simulink model "PubIfDecisionLSM_MDL"  (R2020b)
settings: configuration reference "DspaceConfig" (kept outside this file)
PostLoadFcn:
  | if any(exist('dsrtsu_mdlpostloadfcn', 'file') ~= 0), dsrtsu_mdlpostloadfcn('Execute', bdroot); end
InitFcn:
  | , if any(exist('rtifpga_mdlclblib', 'file') ~= 0), rtifpga_mdlclblib('Init', bdroot); end,
  | , if any(exist('dsmpb_private', 'file') ~= 0), dsmpb_private('dsmpb_mdlclblib', 'Init', bdroot); end,
values from neighbouring files (symbols this model uses):
  P_LSM_ALC_Enable = 0.0    [LSM_Parameter.sldd]
  P_LSM_AwayEdge_offset = 0.1    [LSM_Parameter.sldd]
  P_LSM_CentValidErr = 1.0    [LSM_Parameter.sldd]
  P_LSM_DOP_C0_EN_Limit = 0.8    [LSM_Parameter.sldd]
  P_LSM_DOP_C0_out_Limit = 2.0    [LSM_Parameter.sldd]
  P_LSM_DOP_C1_EN_Limit : value not decoded    [LSM_Parameter.sldd]
  P_LSM_DOP_C1_out_Limit : value not decoded    [LSM_Parameter.sldd]
  P_LSM_DOP_C1AndC2_Lim_X : value not decoded    [LSM_Parameter.sldd]
  P_LSM_DOP_C2_EN_Limit : value not decoded    [LSM_Parameter.sldd]
  P_LSM_DOP_C2_out_Limit : value not decoded    [LSM_Parameter.sldd]
  P_LSM_DOP_In_Pre2Dop_Dis = 1.0    [LSM_Parameter.sldd]
  P_LSM_DOP_Out_Pre2Dop_Dis = 2.0    [LSM_Parameter.sldd]
  P_LSM_DOP_PreDis_X : value not decoded    [LSM_Parameter.sldd]
  P_LSM_DOP_PreDis_Y : value not decoded    [LSM_Parameter.sldd]
  P_LSM_DOPEnableSW = 1.0    [LSM_Parameter.sldd]
  P_LSM_DOPValid_CheckTime = 0.06    [LSM_Parameter.sldd]
  P_LSM_DoubleLine_Curr2Cent_Dislimit = 0.5    [LSM_Parameter.sldd]
  P_LSM_DoubleLine_Dop2Cent_Dislimit = 0.5    [LSM_Parameter.sldd]
  P_LSM_DoubleLine_DOPOut_C1 : value not decoded    [LSM_Parameter.sldd]
  P_LSM_DoubleLine_Pre2Cent_Dislimit = 1.0    [LSM_Parameter.sldd]
  P_LSM_Error_Limit = 0.5    [LSM_Parameter.sldd]
  P_LSM_IFV2CenterAxis = 0.0    [LSM_Parameter.sldd]
  P_LSM_IFV2RearAxis = 0.0    [LSM_Parameter.sldd]
  P_LSM_Line2Edge_limit = 0.5    [LSM_Parameter.sldd]
  P_LSM_Line_Error = 0.1    [LSM_Parameter.sldd]
  P_LSM_LineSTD_Limit = 0.15    [LSM_Parameter.sldd]
  P_LSM_NOH_Switch = 0.0    [LSM_Parameter.sldd]
  P_LSM_OTL_C0_Factor = 1.0    [LSM_Parameter.sldd]
  P_LSM_OTL_C1_Factor = 0.5    [LSM_Parameter.sldd]
  P_LSM_OTL_C2_Factor = 0.5    [LSM_Parameter.sldd]
  P_LSM_Pre2OnlyLineDis = 5.0    [LSM_Parameter.sldd]
  P_LSM_Pre_t = 0.0    [LSM_Parameter.sldd]
  P_LSM_SingleLine_Cent2Edge_Dislimit = 100.0    [LSM_Parameter.sldd]
  P_LSM_SingleLine_Curr2Cent_Dislimit = 0.2    [LSM_Parameter.sldd]
  P_LSM_SingleLine_Dop2Cent_Dislimit = 0.2    [LSM_Parameter.sldd]
  P_LSM_SingleLine_DOPOut_C1 : value not decoded    [LSM_Parameter.sldd]
  P_LSM_SingleLine_Pre2Cent_Dislimit = 0.5    [LSM_Parameter.sldd]
  P_LSM_TJALimitSpd = 60.0    [LSM_Parameter.sldd]
undefined symbols (not defined in the file or in its folder): P_lCS_IFV2CenterAxis, P_LCS_IFV2RearAxis, P_LSM_EntryEdge_offset, P_LSM_EntryLnChngEnSwitch, P_LSM_EntryVanishDis, P_LSM_LinetLostTime, P_LSM_LineWijCal_C12, P_LSM_LineWijCal_C13, P_LSM_MapValid_ErrorSwitch, P_LSM_PosLineLcFac, P_LSM_SpdLim_Stub_Spd, P_LSM_SpdLim_StubLength, P_LSM_SpdTurnAlarm
libraries: simulink x324, TrueDurationTime x11
(part 18 of 25)

== matlab function PubIfDecisionLSM_MDL/Subsystem1/TargetLineCalc_20ms2/TargetLineCalc/CenLineCal1/centerLineFilter ==
  data: LeftLane_change input; RightLane_change input; Line_error input; Edge_error input; Away_offset input; LCKSts input; kap input; preDis input; VisLineConf input uint8 size=4; LineReliable input; VisLineA3 input single size=4; VisLineA2 input single size=4; VisLineA1 input single size=4; VisLineA0 input single size=4; VisLineR input single size=4; VisEdgeConf input uint8 size=2; VisEdgeA3 input single size=2; VisEdgeA2 input single size=2; VisEdgeA1 input single size=2; VisEdgeA0 input single size=2; CentLineConf output boolean size=1; CentLineC3 output single size=1; CentLineC2 output single size=1; CentLineC1 output single size=1; CentLineC0 output single size=1; CentLineRange output single size=1; CenLineReliable output; Line_State output; RoadWidth input; Pre2OnlyLineDis input; Double_Line_Lost output; Offset output; L_CounterK1 input single; R_CounterK1 input single; L_Counter output single; R_Counter output single
function [CentLineConf,CentLineC3,CentLineC2,CentLineC1,CentLineC0,CentLineRange,CenLineReliable,Line_State,Double_Line_Lost,Offset,L_Counter,R_Counter] = ...
    VisFilter(LeftLane_change, RightLane_change, Line_error,Edge_error,Away_offset,LCKSts,kap,preDis,VisLineConf,LineReliable, VisLineA3,VisLineA2,VisLineA1,VisLineA0,VisLineR,...
    VisEdgeConf,VisEdgeA3,VisEdgeA2,VisEdgeA1,VisEdgeA0,RoadWidth,Pre2OnlyLineDis,L_CounterK1,R_CounterK1)
CentLineConf = false;
CentLineC0 = single(0);
CentLineC1 = single(0);
CentLineC2 = single(0);
CentLineC3 = single(0);
CentLineRange = single(0);
CenLineReliable = single(0);
Line_State = uint8(0);
LeftLine2Edg_Error = single(0);
RightLine2Edg_Error = single(0);
Double_Line_Lost = false;
L_Counter = max(L_CounterK1-1,single(0));
R_Counter = max(R_CounterK1-1,single(0));
Left_offset = false;
Right_offset = false;
Left_factor = single(0);
Right_factor = single(0);

dy_pre = 0.5*kap*preDis^2;


Curature2_pre = VisLineA1(2) + 2*VisLineA2(2)*preDis + 3*VisLineA3(2)*(preDis^2);
Curature3_pre = VisLineA1(3) + 2*VisLineA2(3)*preDis + 3*VisLineA3(3)*(preDis^2);
dy2 = (VisLineA0(2) + VisLineA1(2)*preDis + VisLineA2(2)*(preDis^2) + VisLineA3(2)*(preDis^3) - dy_pre)/sqrt(Curature2_pre^2+single(1));
dy3 = (VisLineA0(3) + VisLineA1(3)*preDis + VisLineA2(3)*(preDis^2) + VisLineA3(3)*(preDis^3) - dy_pre)/sqrt(Curature3_pre^2+single(1));
dyLeRE = (VisEdgeA0(1) + VisEdgeA1(1)*preDis + VisEdgeA2(1)*(preDis^2) + VisEdgeA3(1)*(preDis^3) - dy_pre)/sqrt(Curature2_pre^2+single(1));
dyRiRE = (VisEdgeA0(2) + VisEdgeA1(2)*preDis + VisEdgeA2(2)*(preDis^2) + VisEdgeA3(2)*(preDis^3) - dy_pre)/sqrt(Curature3_pre^2+single(1));

%% 边界偏移
if (VisLineConf(2)>=1)&&(VisLineConf(3)>=1)
    if VisEdgeConf(1)>=1&&abs(VisEdgeA0(1)-VisLineA0(2))<Edge_error&&VisEdgeConf(2)>=1&&abs(VisEdgeA0(2)-VisLineA0(3))<Edge_error
        Left_offset = false;
        Right_offset = false;
    elseif VisEdgeConf(1)>=1&&abs(VisEdgeA0(1)-VisLineA0(2))<Edge_error
        Right_offset = true;
    elseif VisEdgeConf(2)>=1&&abs(VisEdgeA0(2)-VisLineA0(3))<Edge_error
        Left_offset = true;
    end
end
if Left_offset
    L_Counter = single(250);
end
if Right_offset
    R_Counter = single(250);
end
if L_Counter>0
    Offset = single(Away_offset);
elseif R_Counter>0
    Offset = single(-Away_offset);
else
    Offset = single(0);
end

%%  限制较宽松
if LCKSts==3
    if (VisLineConf(2)>=1)&&(VisLineConf(3)>=1)
        %         if abs(VisLineA0(2))>Line_error&&abs(VisLineA0(3))>Line_error
        if LeftLane_change==0&&RightLane_change==0
            RoadWidth_Cur = VisLineA0(2)-VisLineA0(3);
            if VisEdgeConf(1)>=1
                LeftLine2Edg_Error = abs(VisEdgeA0(1)-VisLineA0(2)-(dy2-dyLeRE));
            end
            if VisEdgeConf(2)>=1
                RightLine2Edg_Error = abs(VisEdgeA0(2)-VisLineA0(3)-(dy3-dyRiRE));
            end
            
            if RoadWidth_Cur-(dy2-dy3)>0.5                            %前方道路变窄
                if VisEdgeConf(1)>=1&&VisEdgeConf(2)>=1               %双边界存在
                    if LeftLine2Edg_Error<=0.5&&RightLine2Edg_Error<=0.5
                        if dy2+dy3<-0.1
                            CentLineConf = true;
                            CentLineC0 = VisLineA0(2)-0.5*RoadWidth*sqrt(1+VisLineA1(2)*VisLineA1(2)) + Offset;
                            CentLineC1 = VisLineA1(2);
                            CentLineC2 = VisLineA2(2);
                            CentLineC3 = VisLineA3(2);
                            CentLineRange = VisLineR(2);
                            CenLineReliable = LineReliable(2);
                            Line_State = uint8(4);
                        elseif dy2+dy3>0.1
                            CentLineConf = true;
                            CentLineC0 = VisLineA0(3)+0.5*RoadWidth*sqrt(1+VisLineA1(3)*VisLineA1(3)) + Offset;
                            CentLineC1 = VisLineA1(3);
                            CentLineC2 = VisLineA2(3);
                            CentLineC3 = VisLineA3(3);
                            CentLineRange = VisLineR(3);
                            CenLineReliable = LineReliable(3);
                            Line_State = uint8(5);
                        else
                            Range_Error = VisLineR(2) - VisLineR(3);
                            LH1_Offset = single(0.5);
                            LH2_Offset = single(0.5);
                            if Range_Error>10 || Range_Error<-10
                                LH1_Offset = 0.5+min(0.5,Range_Error*0.01);
                                LH2_Offset = 1-LH1_Offset;
                            end
                            Line_State = uint8(6);
                            CentLineConf = true;
                            CentLineC0 = 0.5*(VisLineA0(2) + VisLineA0(3)) + Offset;
                            CentLineC1 = LH1_Offset*VisLineA1(2) + LH2_Offset*VisLineA1(3);
                            CentLineC2 = LH1_Offset*VisLineA2(2) + LH2_Offset*VisLineA2(3);
                            CentLineC3 = LH1_Offset*VisLineA3(2) + LH2_Offset*VisLineA3(3);
                            CentLineRange = max(VisLineR(2),VisLineR(3));
                            CenLineReliable = 0.5*(LineReliable(2)+LineReliable(3));
                        end
                    elseif LeftLine2Edg_Error<=0.5
                        CentLineConf = true;
                        CentLineC0 = VisLineA0(2)-0.5*RoadWidth*sqrt(1+VisLineA1(2)*VisLineA1(2)) + Offset;
                        CentLineC1 = VisLineA1(2);
                        CentLineC2 = VisLineA2(2);
                        CentLineC3 = VisLineA3(2);
                        CentLineRange = VisLineR(2);
                        CenLineReliable = LineReliable(2);
                        Line_State = uint8(7);
                    elseif RightLine2Edg_Error<=0.5
                        CentLineConf = true;
                        CentLineC0 = VisLineA0(3)+0.5*RoadWidth*sqrt(1+VisLineA1(3)*VisLineA1(3)) + Offset;
                        CentLineC1 = VisLineA1(3);
                        CentLineC2 = VisLineA2(3);
                        CentLineC3 = VisLineA3(3);
                        CentLineRange = VisLineR(3);
                        CenLineReliable = LineReliable(3);
                        Line_State = uint8(8);
                    elseif dyLeRE+dyRiRE<-0.5
                        CentLineConf = true;
                        CentLineC0 = VisLineA0(2)-0.5*RoadWidth*sqrt(1+VisLineA1(2)*VisLineA1(2)) + Offset;
                        CentLineC1 = VisLineA1(2);
                        CentLineC2 = VisLineA2(2);
                        CentLineC3 = VisLineA3(2);
                        CentLineRange = VisLineR(2);
                        CenLineReliable = LineReliable(2);
                        Line_State = uint8(7);
                    elseif dyLeRE+dyRiRE>0.5
                        CentLineConf = true;
                        CentLineC0 = VisLineA0(3)+0.5*RoadWidth*sqrt(1+VisLineA1(3)*VisLineA1(3)) + Offset;
                        CentLineC1 = VisLineA1(3);
                        CentLineC2 = VisLineA2(3);
                        CentLineC3 = VisLineA3(3);
                        CentLineRange = VisLineR(3);
                        CenLineReliable = LineReliable(3);
                        Line_State = uint8(8);
                    else
                        Range_Error = VisLineR(2) - VisLineR(3);
                        LH1_Offset = single(0.5);
                        LH2_Offset = single(0.5);
                        if Range_Error>10 || Range_Error<-10
                            LH1_Offset = 0.5+min(0.5,Range_Error*0.01);
                            LH2_Offset = 1-LH1_Offset;
                        end
                        Line_State = uint8(9);
                        CentLineConf = true;
                        CentLineC0 = 0.5*(VisLineA0(2) + VisLineA0(3)) + Offset;
                        CentLineC1 = LH1_Offset*VisLineA1(2) + LH2_Offset*VisLineA1(3);
                        CentLineC2 = LH1_Offset*VisLineA2(2) + LH2_Offset*VisLineA2(3);
                        CentLineC3 = LH1_Offset*VisLineA3(2) + LH2_Offset*VisLineA3(3);
                        CentLineRange = max(VisLineR(2),VisLineR(3));
                        CenLineReliable = 0.5*(LineReliable(2)+LineReliable(3));
                    end
                elseif VisEdgeConf(1)>=1                         %左边界存在
                    CentLineConf = true;
                    CentLineC0 = VisLineA0(2)-0.5*RoadWidth*sqrt(1+VisLineA1(2)*VisLineA1(2)) + Offset;
                    CentLineC1 = VisLineA1(2);
                    CentLineC2 = VisLineA2(2);
                    CentLineC3 = VisLineA3(2);
                    CentLineRange = VisLineR(2);
                    CenLineReliable = LineReliable(2);
                    Line_State = uint8(10);
                elseif VisEdgeConf(2)>=1                         %右边界存在
                    CentLineConf = true;
                    CentLineC0 = VisLineA0(3)+0.5*RoadWidth*sqrt(1+VisLineA1(3)*VisLineA1(3)) + Offset;
                    CentLineC1 = VisLineA1(3);
                    CentLineC2 = VisLineA2(3);
                    CentLineC3 = VisLineA3(3);
                    CentLineRange = VisLineR(3);
                    CenLineReliable = LineReliable(3);
                    Line_State = uint8(11);
                else
                    Range_Error = VisLineR(2) - VisLineR(3);
                    LH1_Offset = single(0.5);
                    LH2_Offset = single(0.5);
                    if Range_Error>10 || Range_Error<-10
                        LH1_Offset = 0.5+min(0.5,Range_Error*0.01);
                        LH2_Offset = 1-LH1_Offset;
                    end
                    Line_State = uint8(12);
                    CentLineConf = true;
                    CentLineC0 = 0.5*(VisLineA0(2) + VisLineA0(3)) + Offset;
                    CentLineC1 = LH1_Offset*VisLineA1(2) + LH2_Offset*VisLineA1(3);
                    CentLineC2 = LH1_Offset*VisLineA2(2) + LH2_Offset*VisLineA2(3);
                    CentLineC3 = LH1_Offset*VisLineA3(2) + LH2_Offset*VisLineA3(3);
                    CentLineRange = max(VisLineR(2),VisLineR(3));
                    CenLineReliable = 0.5*(LineReliable(2)+LineReliable(3));
                end
                
            elseif dy2-dy3-RoadWidth_Cur>0.5                        %前方道路变宽
                %                 if VisEdgeConf(1)>=1&&VisEdgeConf(2)>=1
                %                     if LeftLine2Edg_Error<=0.5&&RightLine2Edg_Error<=0.5
                %                         if dy2+dy3<-0.1
                %                             CentLineConf = true;
                %                             CentLineC0 = VisLineA0(2)-0.5*RoadWidth*sqrt(1+VisLineA1(2)*VisLineA1(2)) + Offset;
                %                             CentLineC1 = VisLineA1(2);
                %                             CentLineC2 = VisLineA2(2);
                %                             CentLineC3 = VisLineA3(2);
                %                             CentLineRange = VisLineR(2);
                %                             Line_State = uint8(13);
                %                         elseif dy2+dy3>0.1
                %                             CentLineConf = true;
                %                             CentLineC0 = VisLineA0(3)+0.5*RoadWidth*sqrt(1+VisLineA1(3)*VisLineA1(3)) + Offset;
                %                             CentLineC1 = VisLineA1(3);
                %                             CentLineC2 = VisLineA2(3);
                %                             CentLineC3 = VisLineA3(3);
                %                             CentLineRange = VisLineR(3);
                %                             Line_State = uint8(14);
                %                         else
                %                             Range_Error = VisLineR(2) - VisLineR(3);
                %                             LH1_Offset = single(0.5);
                %                             LH2_Offset = single(0.5);
                %                             if Range_Error>10 || Range_Error<-10
                %                                 LH1_Offset = 0.5+min(0.5,Range_Error*0.01);
                %                                 LH2_Offset = 1-LH1_Offset;
                %                             end
                %                             Line_State = uint8(15);
                %                             CentLineConf = true;
                %                             CentLineC0 = 0.5*(VisLineA0(2) + VisLineA0(3)) + Offset;
                %                             CentLineC1 = LH1_Offset*VisLineA1(2) + LH2_Offset*VisLineA1(3);
                %                             CentLineC2 = LH1_Offset*VisLineA2(2) + LH2_Offset*VisLineA2(3);
                %                             CentLineC3 = LH1_Offset*VisLineA3(2) + LH2_Offset*VisLineA3(3);
                %                             CentLineRange = max(VisLineR(2),VisLineR(3));
                %                         end
                %                     elseif LeftLine2Edg_Error<=0.5
                %                         CentLineConf = true;
                %                         CentLineC0 = VisLineA0(2)-0.5*RoadWidth*sqrt(1+VisLineA1(2)*VisLineA1(2)) + Offset;
                %                         CentLineC1 = VisLineA1(2);
                %                         CentLineC2 = VisLineA2(2);
                %                         CentLineC3 = VisLineA3(2);
                %                         CentLineRange = VisLineR(2);
                %                         Line_State = uint8(16);
                %                     elseif RightLine2Edg_Error<=0.5
                %                         CentLineConf = true;
                %                         CentLineC0 = VisLineA0(3)+0.5*RoadWidth*sqrt(1+VisLineA1(3)*VisLineA1(3)) + Offset;
                %                         CentLineC1 = VisLineA1(3);
                %                         CentLineC2 = VisLineA2(3);
                %                         CentLineC3 = VisLineA3(3);
                %                         CentLineRange = VisLineR(3);
                %                         Line_State = uint8(17);
                %                     else
                %                         Range_Error = VisLineR(2) - VisLineR(3);
                %                         LH1_Offset = single(0.5);
                %                         LH2_Offset = single(0.5);
                %                         if Range_Error>10 || Range_Error<-10
                %                             LH1_Offset = 0.5+min(0.5,Range_Error*0.01);
                %                             LH2_Offset = 1-LH1_Offset;
                %                         end
                %                         Line_State = uint8(18);
                %                         CentLineConf = true;
                %                         CentLineC0 = 0.5*(VisLineA0(2) + VisLineA0(3)) + Offset;
                %                         CentLineC1 = LH1_Offset*VisLineA1(2) + LH2_Offset*VisLineA1(3);
                %                         CentLineC2 = LH1_Offset*VisLineA2(2) + LH2_Offset*VisLineA2(3);
                %                         CentLineC3 = LH1_Offset*VisLineA3(2) + LH2_Offset*VisLineA3(3);
                %                         CentLineRange = max(VisLineR(2),VisLineR(3));
                %                     end
                %                     %         elseif VisEdgeConf(1)>=1                         %左边界存在
                %                     %             CentLineConf = true;
                %                     %             CentLineC0 = VisLineA0(2)-0.5*RoadWidth*sqrt(1+VisLineA1(2)*VisLineA1(2));
                %                     %             CentLineC1 = VisLineA1(2);
                %                     %             CentLineC2 = VisLineA2(2);
                %                     %             CentLineC3 = VisLineA3(2);
                %                     %             CentLineRange = VisLineR(2);
                %                     %             Line_State = uint8(19);
                %                     %         elseif VisEdgeConf(2)>=1                         %右边界存在
                %                     %             CentLineConf = true;
                %                     %             CentLineC0 = VisLineA0(3)+0.5*RoadWidth*sqrt(1+VisLineA1(3)*VisLineA1(3));
                %                     %             CentLineC1 = VisLineA1(3);
                %                     %             CentLineC2 = VisLineA2(3);
                %                     %             CentLineC3 = VisLineA3(3);
                %                     %             CentLineRange = VisLineR(3);
                %                     %             Line_State = uint8(20);
                %                     %         else
                %                     %             Range_Error = VisLineR(2) - VisLineR(3);
                %                     %             LH1_Offset = single(0.5);
                %                     %             LH2_Offset = single(0.5);
                %                     %             if Range_Error>10 || Range_Error<-10
                %                     %                 LH1_Offset = 0.5+min(0.5,Range_Error*0.01);
                %                     %                 LH2_Offset = 1-LH1_Offset;
                %                     %             end
                %                     %             Line_State = uint8(21);
                %                     %             CentLineConf = true;
                %                     %             CentLineC0 = 0.5*(VisLineA0(2) + VisLineA0(3));
                %                     %             CentLineC1 = LH1_Offset*VisLineA1(2) + LH2_Offset*VisLineA1(3);
                %                     %             CentLineC2 = LH1_Offset*VisLineA2(2) + LH2_Offset*VisLineA2(3);
                %                     %             CentLineC3 = LH1_Offset*VisLineA3(2) + LH2_Offset*VisLineA3(3);
                %                     %             CentLineRange = max(VisLineR(2),VisLineR(3));
                %                     %         end
                %                 else
                if dy2+dy3<-0.1
                    CentLineConf = true;
                    CentLineC0 = VisLineA0(2)-0.5*RoadWidth*sqrt(1+VisLineA1(2)*VisLineA1(2)) + Offset;
                    CentLineC1 = VisLineA1(2);
                    CentLineC2 = VisLineA2(2);
                    CentLineC3 = VisLineA3(2);
                    CentLineRange = VisLineR(2);
                    CenLineReliable = LineReliable(2);
                    Line_State = uint8(19);
                elseif dy2+dy3>0.1
                    CentLineConf = true;
                    CentLineC0 = VisLineA0(3)+0.5*RoadWidth*sqrt(1+VisLineA1(3)*VisLineA1(3)) + Offset;
                    CentLineC1 = VisLineA1(3);
                    CentLineC2 = VisLineA2(3);
                    CentLineC3 = VisLineA3(3);
                    CentLineRange = VisLineR(3);
                    CenLineReliable = LineReliable(3);
                    Line_State = uint8(20);
                else
                    Range_Error = VisLineR(2) - VisLineR(3);
                    LH1_Offset = single(0.5);
                    LH2_Offset = single(0.5);
                    if Range_Error>10 || Range_Error<-10
                        LH1_Offset = 0.5+min(0.5,Range_Error*0.01);
                        LH2_Offset = 1-LH1_Offset;
                    end
                    Line_State = uint8(22);
                    CentLineConf = true;
                    CentLineC0 = 0.5*(VisLineA0(2) + VisLineA0(3)) + Offset;
                    CentLineC1 = LH1_Offset*VisLineA1(2) + LH2_Offset*VisLineA1(3);
                    CentLineC2 = LH1_Offset*VisLineA2(2) + LH2_Offset*VisLineA2(3);
                    CentLineC3 = LH1_Offset*VisLineA3(2) + LH2_Offset*VisLineA3(3);
                    CentLineRange = max(VisLineR(2),VisLineR(3));
                    CenLineReliable = 0.5*(LineReliable(2)+LineReliable(3));
                end
            else
                temp = (VisLineA0(2) - VisLineA0(3))/sqrt(VisLineA1(2)^2 + single(1));
                if temp>4.2
                    if abs(VisLineA0(2))>abs(VisLineA0(3))
                        CentLineConf = true;
                        CentLineC0 = VisLineA0(3)+0.5*RoadWidth*sqrt(1+VisLineA1(3)*VisLineA1(3)) + Offset;
                        CentLineC1 = VisLineA1(3);
                        CentLineC2 = VisLineA2(3);
                        CentLineC3 = VisLineA3(3);
                        CentLineRange = VisLineR(3);
                        CenLineReliable = LineReliable(3);
                        Line_State = uint8(23);
                    elseif abs(VisLineA0(2))<=abs(VisLineA0(3))
                        CentLineConf = true;
                        CentLineC0 = VisLineA0(2)-0.5*RoadWidth*sqrt(1+VisLineA1(2)*VisLineA1(2)) + Offset;
                        CentLineC1 = VisLineA1(2);
                        CentLineC2 = VisLineA2(2);
                        CentLineC3 = VisLineA3(2);
                        CentLineRange = VisLineR(2);
                        CenLineReliable = LineReliable(2);
                        Line_State = uint8(23);
                    end
                else
                    Range_Error = VisLineR(2) - VisLineR(3);
                    LH1_Offset = single(0.5);
                    LH2_Offset = single(0.5);
                    if Range_Error>10 || Range_Error<-10
                        LH1_Offset = 0.5+min(0.5,Range_Error*0.01);
                        LH2_Offset = 1-LH1_Offset;
                    end
                    Line_State = uint8(23);
                    CentLineConf = true;
                    CentLineC0 = 0.5*(VisLineA0(2) + VisLineA0(3)) + Offset;
                    CentLineC1 = LH1_Offset*VisLineA1(2) + LH2_Offset*VisLineA1(3);
                    CentLineC2 = LH1_Offset*VisLineA2(2) + LH2_Offset*VisLineA2(3);
                    CentLineC3 = LH1_Offset*VisLineA3(2) + LH2_Offset*VisLineA3(3);
                    CentLineRange = max(VisLineR(2),VisLineR(3));
                    CenLineReliable = 0.5*(LineReliable(2)+LineReliable(3));
                end
            end
        end
    elseif VisLineConf(2)>=1                    %只存在左侧线
        if VisEdgeConf(2)>=1
            LeftLine_Edge_Width = (VisLineA0(2) - VisEdgeA0(2))/sqrt(VisLineA1(2)^2 + single(1));
            if LeftLine_Edge_Width>=2.6 && abs(dy2)<Pre2OnlyLineDis
                CentLineConf = true;
                CentLineC0 = VisLineA0(2)-min(RoadWidth,LeftLine_Edge_Width)*0.5*sqrt(1+VisLineA1(2)*VisLineA1(2))+Offset;
                CentLineC1 = VisLineA1(2);
                CentLineC2 = VisLineA2(2);
                CentLineC3 = VisLineA3(2);
                CentLineRange = VisLineR(2);
                CenLineReliable = LineReliable(2);
                Line_State = uint8(24);
            end
        else
            if abs(VisLineA0(2))>Line_error
                CentLineConf = true;
                CentLineC0 = VisLineA0(2)-0.5*RoadWidth*sqrt(1+VisLineA1(2)*VisLineA1(2));
                CentLineC1 = VisLineA1(2);
                CentLineC2 = VisLineA2(2);
                CentLineC3 = VisLineA3(2);
                CentLineRange = VisLineR(2);
                CenLineReliable = LineReliable(2);
                Line_State = uint8(24);
            end
        end
        
    elseif VisLineConf(3)>=1              %只存在右侧线
        if VisEdgeConf(1)>=1
            RightLine_Edge_Width = (VisEdgeA0(1)-VisLineA0(3))/sqrt(VisLineA1(3)^2 + single(1));
            if RightLine_Edge_Width>=2.6 && abs(dy3)<Pre2OnlyLineDis
                CentLineConf = true;
                CentLineC0 = VisLineA0(3)+min(RoadWidth,RightLine_Edge_Width)*0.5*sqrt(1+VisLineA1(3)*VisLineA1(3))+Offset;
                CentLineC1 = VisLineA1(3);
                CentLineC2 = VisLineA2(3);
                CentLineC3 = VisLineA3(3);
                CentLineRange = VisLineR(3);
                CenLineReliable = LineReliable(3);
                Line_State = uint8(25);
            end
        else
            if abs(VisLineA0(3))>Line_error
                CentLineConf = true;
                CentLineC0 = VisLineA0(3)+0.5*RoadWidth*sqrt(1+VisLineA1(3)*VisLineA1(3));
                CentLineC1 = VisLineA1(3);
                CentLineC2 = VisLineA2(3);
                CentLineC3 = VisLineA3(3);
                CentLineRange = VisLineR(3);
                CenLineReliable = 0.5*(LineReliable(2)+LineReliable(3));
                Line_State = uint8(25);
            end
        end
    else
        Double_Line_Lost = true;
    end
    %%   限制增加
else
    if (VisLineConf(2)>1)&&(VisLineConf(3)>1)&&...        %  0.04  ~~~2.5
            (VisLineR(2)>20||VisLineR(3)>20)&&...
            (abs(0.5*VisLineA0(2) + 0.5*VisLineA0(3))<2)&&....
            RoadWidth>=2.5&&RoadWidth<=5&&abs(VisLineA0(2))>0.2&&abs(VisLineA0(3))>0.2&&...
            (dy2-dy3)>=2&&(dy2-dy3)<=5.5
        
        Range_Error = VisLineR(2) - VisLineR(3);
        LH1_Offset = single(0.5);
        LH2_Offset = single(0.5);
        Line_State = uint8(1);
        if Range_Error>10 || Range_Error<-10
            LH1_Offset = 0.5+min(0.5,Range_Error*0.01);
            LH2_Offset = 1-LH1_Offset;
        end
        CentLineConf = true;
        CentLineC0 = 0.5*(VisLineA0(2) + VisLineA0(3))+Offset;
        CentLineC1 = LH1_Offset*VisLineA1(2) + LH2_Offset*VisLineA1(3);
        CentLineC2 = LH1_Offset*VisLineA2(2) + LH2_Offset*VisLineA2(3);
        CentLineC3 = LH1_Offset*VisLineA3(2) + LH2_Offset*VisLineA3(3);
        CentLineRange = max(VisLineR(2),VisLineR(3));
        CenLineReliable = 0.5*(LineReliable(2)+LineReliable(3));
        
    elseif VisLineConf(2)>1&&VisLineR(2)>20&&...             %单左侧
            VisLineA0(2)>0.3*RoadWidth&&...
            VisLineA0(2)<0.7*RoadWidth&&...
            dy2>0.2*RoadWidth && dy2<0.9*RoadWidth
            
        if VisEdgeConf(2)>=1
            LeftLine_Edge_Width = (VisLineA0(2) - VisEdgeA0(2))/sqrt(VisLineA1(2)^2 + single(1));
            if LeftLine_Edge_Width>=3
                CentLineConf = true;
                CentLineC0 = VisLineA0(2)-min(LeftLine_Edge_Width,RoadWidth)*0.5*sqrt(1+VisLineA1(2)*VisLineA1(2))+Offset;
                CentLineC1 = VisLineA1(2);
                CentLineC2 = VisLineA2(2);
                CentLineC3 = VisLineA3(2);
                CentLineRange = VisLineR(2);
                CenLineReliable = LineReliable(2);
                Line_State = uint8(2);
            end
        else
            Line_State = uint8(2);
            CentLineConf = true;
            CentLineC0 = VisLineA0(2) - 0.5*RoadWidth*sqrt(1+VisLineA1(2)*VisLineA1(2));
            CentLineC1 = VisLineA1(2);
            CentLineC2 = VisLineA2(2);
            CentLineC3 = VisLineA3(2);
            CentLineRange = VisLineR(2);
            CenLineReliable = LineReliable(2);
        end
        
    elseif VisLineConf(3)>1&&VisLineR(3)>20&&...      %单右侧
            VisLineA0(3)<-0.3*RoadWidth&&...
            VisLineA0(3)>-0.7*RoadWidth&&...
            dy3<-0.2*RoadWidth && dy3>-0.9*RoadWidth
        if VisEdgeConf(1)>=1
            RightLine_Edge_Width = (VisEdgeA0(1)-VisLineA0(3))/sqrt(VisLineA1(3)^2 + single(1));
            if RightLine_Edge_Width>=3
                CentLineConf = true;
                CentLineC0 = VisLineA0(3)+min(RightLine_Edge_Width,RoadWidth)*0.5*sqrt(1+VisLineA1(3)*VisLineA1(3))+Offset;
                CentLineC1 = VisLineA1(3);
                CentLineC2 = VisLineA2(3);
                CentLineC3 = VisLineA3(3);
                CentLineRange = VisLineR(3);
                CenLineReliable = LineReliable(3);
                Line_State = uint8(3);
            end
        else
            Line_State = uint8(3);
            CentLineConf = true;
            CentLineC0 = VisLineA0(3) + 0.5*RoadWidth*sqrt(1+VisLineA1(3)*VisLineA1(3));
            CentLineC1 = VisLineA1(3);
            CentLineC2 = VisLineA2(3);
            CentLineC3 = VisLineA3(3);
            CentLineRange = VisLineR(3);
            CenLineReliable = LineReliable(3);
        end
    end
end
end
